simulink model "Imbardata"  (Simulink 8.5)
settings: Solver=ode1  StartTime=0.0  StopTime=200  RelTol=1e-3
libraries: simulink x1
settings Model: Creator=Pera  LastModifiedBy=alastor  CovSFcnEnable=off
settings DataIOCC: SignalLoggingSaveFormat=Dataset
settings OptimizationCC: ExpressionDepthLimit=128
settings DebuggingCC: SolverPrmCheckMsg=warning  FcnCallInpInsideContextMsg=EnableAllAsError
settings HardwareCC: ProdLargestAtomicInteger=Long  ProdLargestAtomicFloat=Double  ProdIntDivRoundTo=Floor  ProdEndianess=LittleEndian  ProdHWDeviceType=ARM Compatible->ARM Cortex
settings RTWCC: GenCodeOnly=on  PackageGeneratedCodeAndArtifacts=on  PackageName=prova  GenerateReport=on  LaunchReport=on  TargetLang=C++
settings GRTTargetCC: CombineOutputUpdateFcns=on  MatFileLogging=off  MultiInstanceERTCode=on  CodeInterfacePackaging=C++ class  GRTInterface=off
settings CPPComponent: GenerateDestructor=on  GenerateExternalIOAccessMethods=None  ParameterMemberVisibility=private  InternalMemberVisibility=private  GenerateParameterAccessMethods=None  GenerateInternalMemberAccessMethods=None  UseOperatorNewForModelRefRegistration=off

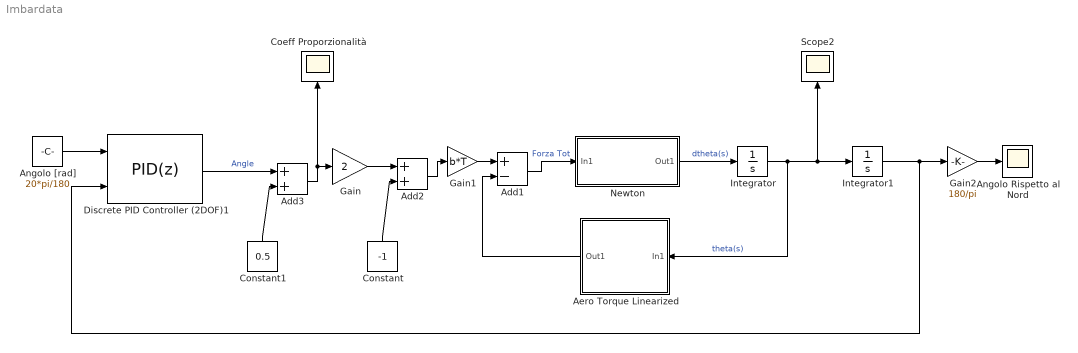
== system Imbardata ==
  Add1 : Sum  Inputs=+-
  Add2 : Sum
  Add3 : Sum
  Aero Torque Linearized : Subsystem  mask{rho=1.225, radius=0.4, cd=0.5, d=0.5}
      mask prompts: rho "density"; cd "drag coeff"; d "baricentro-centro pallone"
      mask init:
      | s1=['rho= ',num2str(rho)];
      | s2=['radius= ',num2str(radius)];
      | s3=['cd= ',num2str(cd)];
      | s4=['d= ',num2str(d)];
      | s=strvcat(s1,s2,s3,s4);  %sto concatenando verticalmente
      mask Display: disp(s)
  Angolo Rispetto al Nord : Scope
  Angolo [rad] : Constant  Value=20*pi/180
  Coeff Proporzionalità : Scope
      settings: MaxDataPoints=10000
  Constant : Constant  Value=-1
  Constant1 : Constant  Value=0.5
  Discrete PID Controller (2DOF)1 : simulink/Continuous/PID Controller (2DOF)  Controller=PID  TimeDomain=Discrete-time  SampleTime=0.5  IntegratorMethod=Forward Euler  FilterMethod=Forward Euler  Form=Parallel  UseFilter=on  ControllerParametersSource=internal  P=0.172446391413693  I=0.000376633033333102  D=0.185232201612025  N=3.50932224937588  b=1  c=1  InitialConditionSource=internal  InitialConditionForIntegrator=0  InitialConditionForFilter=0  ExternalReset=none  LimitOutput=on  UpperSaturationLimit=0.5  LowerSaturationLimit=-0.5  LinearizeAsGain=off  AntiWindupMode=back-calculation  Kb=1  TrackingMode=off  Kt=1  PParamMin=[]  PParamMax=[]  IParamMin=[]  IParamMax=[]  DParamMin=[]  DParamMax=[]  NParamMin=[]  NParamMax=[]  bParamMin=[]  bParamMax=[]  cParamMin=[]  cParamMax=[]  KbParamMin=[]  KbParamMax=[]  KtParamMin=[]  KtParamMax=[]  POutMin=[]  POutMax=[]  IOutMin=[]  IOutMax=[]  DOutMin=[]  DOutMax=[]  NOutMin=[]  NOutMax=[]  bOutMin=[]  bOutMax=[]  cOutMin=[]  cOutMax=[]  KbOutMin=[]  KbOutMax=[]  KtOutMin=[]  KtOutMax=[]  IntegratorOutMin=[]  IntegratorOutMax=[]  FilterOutMin=[]  FilterOutMax=[]  SumOutMin=[]  SumOutMax=[]  Sum1OutMin=[]  Sum1OutMax=[]  Sum2OutMin=[]  Sum2OutMax=[]  Sum3OutMin=[]  Sum3OutMax=[]  SumI1OutMin=[]  SumI1OutMax=[]  SumI2OutMin=[]  SumI2OutMax=[]  SumI3OutMin=[]  SumI3OutMax=[]  SumDOutMin=[]  SumDOutMax=[]  SaturationOutMin=[]  SaturationOutMax=[]  IntegratorContinuousStateAttributes=''  IntegratorStateMustResolveToSignalObject=off  IntegratorRTWStateStorageClass=Auto  FilterContinuousStateAttributes=''  FilterStateMustResolveToSignalObject=off  FilterRTWStateStorageClass=Auto  DifferentiatorICPrevScaledInput=0  DifferentiatorOutMin=[]  DifferentiatorOutMax=[]
  Gain : Gain  Gain=2
  Gain1 : Gain  Gain=b*T  mask{b=0.4, T=0.3}
      mask prompts: b "braccio [m]"; T "thrust [N]"
  Gain2 : Gain  Gain=180/pi
  Integrator : Integrator
  Integrator1 : Integrator
  Newton : Subsystem  mask{J=0.3}
      mask prompts: J "Inertia"
      mask init:
      | s=['Inertia= ',num2str(J),' [Kg*m^2]'];
      mask Display: disp(s)
  Scope2 : Scope
      settings: SaveName=ScopeData2  MaxDataPoints=10000
  wires:
  Newton/1(Out1) -> Integrator/1  "dtheta(s)"
  Integrator/1 -> Aero Torque Linearized/1(In1), Integrator1/1, Scope2/1  "theta(s)"
  Add1/1 -> Newton/1(In1)  "Forza Tot"
  Aero Torque Linearized/1(Out1) -> Add1/2
  Angolo [rad]/1 -> Discrete PID Controller (2DOF)1/1
  Integrator1/1 -> Discrete PID Controller (2DOF)1/2, Gain2/1
  Gain/1 -> Add2/1
  Constant/1 -> Add2/2
  Gain1/1 -> Add1/1
  Add2/1 -> Gain1/1
  Gain2/1 -> Angolo Rispetto al Nord/1
  Discrete PID Controller (2DOF)1/1 -> Add3/1  "Angle"
  Add3/1 -> Coeff Proporzionalità/1, Gain/1
  Constant1/1 -> Add3/2

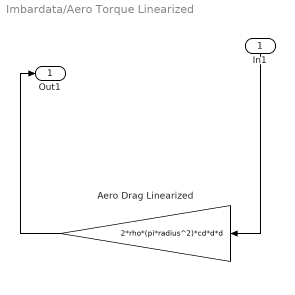
== system Imbardata/Aero Torque Linearized ==
  In1 : Inport
  Aero Drag Linearized : Gain  Gain=2*rho*(pi*radius^2)*cd*d*d
  Out1 : Outport
  wires:
  In1/1 -> Aero Drag Linearized/1
  Aero Drag Linearized/1 -> Out1/1

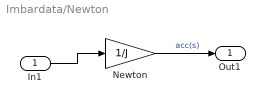
== system Imbardata/Newton ==
  In1 : Inport
  Newton : Gain  Gain=1/J
  Out1 : Outport
  wires:
  In1/1 -> Newton/1
  Newton/1 -> Out1/1  "acc(s)"
